simulink model "thingg"  (R2015a)
settings: Solver=ode45  StartTime=0.0  StopTime=10.0  RelTol=1e-3
settings Model: Creator=STEM Student  LastModifiedBy=STEM Student

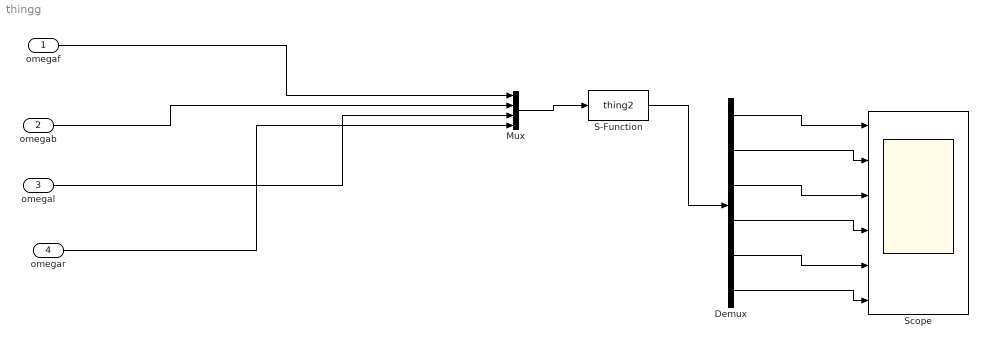
== system thingg ==
  omegaf : Inport
  omegab : Inport  Port=2
  omegal : Inport  Port=3
  omegar : Inport  Port=4
  Demux : Demux  Outputs=6
  Mux : Mux
  S-Function : S-Function  FunctionName=thing2
  Scope : Scope  NumInputPorts=6
      settings: YMin=-5~-5~-5~-5~-5~-5  YMax=5~5~5~5~5~5
  wires:
  omegaf/1 -> Mux/1
  omegab/1 -> Mux/2
  omegal/1 -> Mux/3
  omegar/1 -> Mux/4
  Mux/1 -> S-Function/1
  S-Function/1 -> Demux/1
  Demux/1 -> Scope/1
  Demux/2 -> Scope/2
  Demux/3 -> Scope/3
  Demux/4 -> Scope/4
  Demux/5 -> Scope/5
  Demux/6 -> Scope/6
